simulink model "Simulacion_b"  (R2021a)
settings: Solver=ode4  StartTime=0.0  StopTime=500  FixedStep=0.01  RelTol=1e-3
values from neighbouring files (symbols this model uses):
  Qi = 8/(1000*60)    (= 0.000133333333333)    [TP1.m]
  ue = double(ue)    [TP1.m]
  x1e = 0.45    [TP1.m]
  ye = 0.45    [TP1.m]
libraries: cstblocks x3
settings Model: Creator=amddy  LastModifiedBy=Usuario

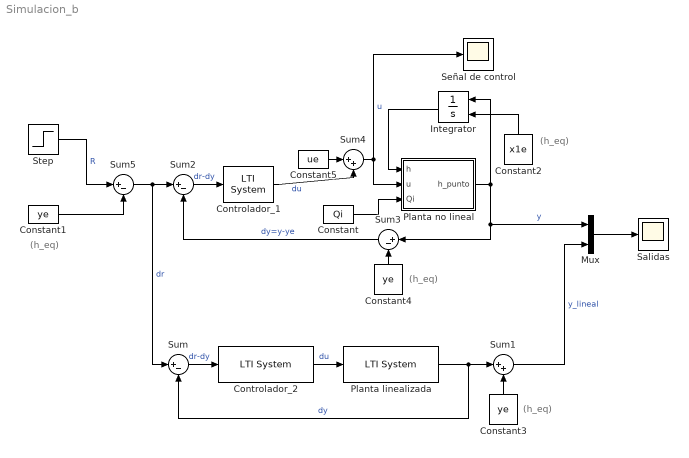
== system Simulacion_b ==
  note: (h_eq)
  note: (h_eq)
  note: (h_eq)
  note: (h_eq)
  Constant : Constant  Value=Qi
  Constant1 : Constant  Value=ye
  Constant2 : Constant  Value=x1e
  Constant3 : Constant  Value=ye
  Constant4 : Constant  Value=ye
  Constant5 : Constant  Value=ue
  Controlador_1 : cstblocks/LTI System  sys=C  IC=[]
  Controlador_2 : cstblocks/LTI System  sys=C  IC=[]
  Integrator : Integrator  InitialConditionSource=external
  Mux : Mux  Inputs=2
  Planta linealizada : cstblocks/LTI System  sys=G  IC=[]
  Planta no lineal : MATLAB Function  TreatAsAtomicUnit=on
  Salidas : Scope
  Señal de control : Scope
  Step : Step  Time=0  After=0.55  SampleTime=0
  Sum{,2..3,5} (4 alike) : Sum  Inputs=|+-
  Sum1 : Sum  Inputs=|++
  Sum4 : Sum  Inputs=|++
  wires:
  Integrator/1 -> Planta no lineal/1(h)
  Constant/1 -> Planta no lineal/3(Qi)
  Planta no lineal/1(h_punto) -> Mux/1, Sum3/1, Integrator/1  "y"
  Mux/1 -> Salidas/1
  Constant2/1 -> Integrator/2
  Planta linealizada/1 -> Sum/2, Sum1/1  "dy"
  Sum1/1 -> Mux/2  "y_lineal"
  Constant3/1 -> Sum1/2
  Sum/1 -> Controlador_2/1  "dr-dy"
  Controlador_2/1 -> Planta linealizada/1  "du"
  Sum2/1 -> Controlador_1/1  "dr-dy"
  Sum3/1 -> Sum2/2  "dy=y-ye"
  Constant4/1 -> Sum3/2
  Constant5/1 -> Sum4/1
  Sum4/1 -> Planta no lineal/2(u), Señal de control/1  "u"
  Sum5/1 -> Sum/1, Sum2/1  "dr"
  Step/1 -> Sum5/1  "R"
  Constant1/1 -> Sum5/2
  Controlador_1/1 -> Sum4/2  "du"

== matlab function Simulacion_b/Planta no lineal ==
  data: h input; h_punto output; u input; Qi input
function h_punto  = fcn(h,u,Qi)

d_tuberia= 10.65e-3; % metros
lb = 10e-2;  % metros
la= 40e-2; % metros
S= pi*((d_tuberia/2)^2); % metros^2
L=0.9; % metros
g=9.81; % metros/seg^2

h_punto= (Qi - S*u*sqrt(2*g*h))/(lb + (la - lb)*h/L);
end
